simulink model "rtwdemo_cgv"  (Simulink 7.6)
settings: Solver=FixedStepDiscrete  StartTime=0.0  StopTime=10  FixedStep=0.1  RelTol=1e-3
PostLoadFcn:
  | rtwdemo_cgv_init;
  | load('rtwdemo_cgv_data');
values from neighbouring files (symbols this model uses):
  K1 = 3    [rtwdemo_cgv_init.m]    (also in rtwdemo_dow_data.m)
  K2 = 4    [rtwdemo_cgv_init.m]
  K3 = 2.7    [rtwdemo_cgv_init.m]
  Seed = round(cputime*1000)    [rtwdemo_cgv_init.m]
Description:
  | Using Code Generation Verification (CGV)
  | This model is used by the rtwdemo_cgv_script to show CGV Configuration,
  | execution, and comparison support.
settings Model: Creator=The MathWorks Inc.
settings DataIOCC: ExternalInput=BusInput1, upcount, pops, arraySig  LimitDataPoints=off  LoadExternalInput=on  SaveFormat=StructureWithTime  SaveOutput=off  SaveTime=off
settings OptimizationCC: InlineParams=on  InlineInvariantSignals=on  PassReuseOutputArgsAs=Individual arguments  ZeroExternalMemoryAtStartup=off  ZeroInternalMemoryAtStartup=off  EfficientFloat2IntCast=on  OptimizeModelRefInitCode=on  LifeSpan=1
settings DebuggingCC: UnderspecifiedInitializationDetection=Simplified  MergeDetectMultiDrivingBlocksExec=error
settings HardwareCC: ProdIntDivRoundTo=Zero  ProdEndianess=LittleEndian  ProdHWDeviceType=Specified
settings RTWCC: SystemTargetFile=ert.tlc  TemplateMakefile=ert_default_tmf  Description=Real-Time Workshop Embedded Coder  RTWVerbose=off  ProcessScript=ert_make_rtw_hook
settings CodeAppCC: IgnoreCustomStorageClasses=off  IgnoreTestpoints=on
settings ERTTargetCC: MultiwordLength=2048  GenerateSampleERTMain=on  SupportContinuousTime=on  ERTCustomFileTemplate=example_file_process.tlc  ERTFilePackagingFormat=CompactWithDataFile  ConvertIfToSwitch=off

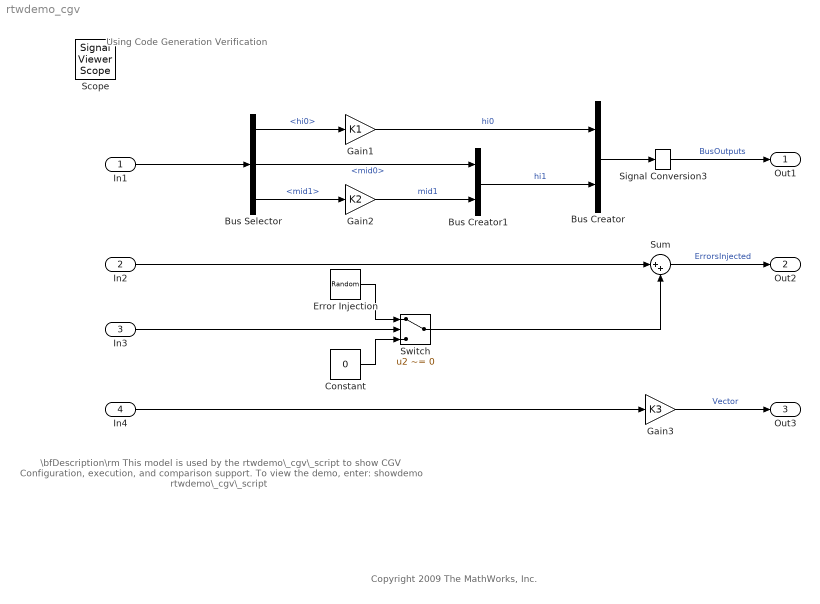
== system rtwdemo_cgv ==
  note: Using Code Generation Verification
  note: \bfDescription\rm
      | This model is used by the rtwdemo\_cgv\_script to show CGV Configuration,
      | execution, and comparison support.  To view the demo, enter:
      | showdemo rtwdemo\_cgv\_script
  note: Copyright 2009 The MathWorks, Inc.
  In1 : Inport  OutDataTypeStr=Bus: TopBus  Interpolate=off
  In2 : Inport  Port=2  OutDataTypeStr=double  PortDimensions=1  SampleTime=.1
  In3 : Inport  Port=3  OutDataTypeStr=double  PortDimensions=1  SampleTime=.1
  In4 : Inport  Port=4  OutDataTypeStr=double  PortDimensions=4  SampleTime=.1
  Bus Creator : BusCreator  Inputs=2  OutDataTypeStr=Bus: TopBus
  Bus Creator1 : BusCreator  Inputs=2  OutDataTypeStr=Bus: MidBus
  Bus Selector : BusSelector  OutputSignals=hi0,hi1.mid0,hi1.mid1
  Constant : Constant  Value=0
  Error Injection : RandomNumber  Variance=.5  Seed=Seed  SampleTime=.1
  Gain1 : Gain  Gain=K1  OutDataTypeStr=Inherit: Same as input
  Gain2 : Gain  Gain=K2  OutDataTypeStr=Inherit: Same as input
  Gain3 : Gain  Gain=K3  OutDataTypeStr=Inherit: Same as input
  Signal Conversion3 : SignalConversion  ConversionOutput=Nonvirtual bus
  Sum : Sum  Inputs=|++
  Switch : Switch  Criteria=u2 ~= 0  Threshold=1
  Out1 : Outport  OutDataTypeStr=Bus: TopBus  BusOutputAsStruct=on
  Out2 : Outport  Port=2
  Out3 : Outport  Port=3
  Scope : SignalViewerScope  IOType=viewer  NumInputPorts=3  RefreshTime=0.035000
      settings: YMin=-5~-5~-5  YMax=5~5~5
  wires:
  In2/1 -> Sum/1
  Sum/1 -> Out2/1  "ErrorsInjected"
  In1/1 -> Bus Selector/1
  Bus Creator/1 -> Signal Conversion3/1
  Bus Selector/2 -> Bus Creator1/1  "<mid0>"
  Bus Selector/1 -> Gain1/1  "<hi0>"
  Bus Selector/3 -> Gain2/1  "<mid1>"
  Gain2/1 -> Bus Creator1/2  "mid1"
  In4/1 -> Gain3/1
  Gain1/1 -> Bus Creator/1  "hi0"
  Bus Creator1/1 -> Bus Creator/2  "hi1"
  Signal Conversion3/1 -> Out1/1  "BusOutputs"
  In3/1 -> Switch/2
  Switch/1 -> Sum/2
  Error Injection/1 -> Switch/1
  Constant/1 -> Switch/3
  Gain3/1 -> Out3/1  "Vector"
